simulink model "Gewerk2_Bahnplanung2015"  (Simulink 8.6)
settings: Solver=ode3  StartTime=0.0  StopTime=inf  FixedStep=0.005  RelTol=1e-3
undefined symbols (not defined in the file or in its folder): Com1, none
libraries: xpcrtudplib x9, xpcutilitieslib x5, xpcseriallib x1, slrtlib x1
(part 2 of 2)

== stateflow chart Gewerk2/Chart ==
  state ?
    state Hauptprogramm [parallel]
      settings: executionOrder=1
      state Auftrag_Roboter_1
      state Zielbereich_untersuchen
        entry:
        n4=round((Robbi4_x-528)/400);
        n2=round((Robbi2_x-528)/400);
        n3=round((Robbi3_x-528)/400);
        y2=Robbi2_y;
        y3=Robbi3_y;
        y4=Robbi4_y;
        ersterFifo=floor(Zielstationstation/2)*3+2*mod(Zielstation,2);
      state Uebergabepunkt_gleich_Zielpunkt
        entry:
        for i=1:1:8
        Fifo(i)=0;
        end
        Vektorberechnung=1;
        Auftragskoordinaten=Zielpostion;
      state Fifo_besetzt
        entry:
        Fifobelegt=1;
        zweiterFifo=floor(Zielstation/2)*3+1;
      state Fifo_doppelt_besetzt
        entry:
        dritterFifo=floor(Zielstation/2)*3+2-2*mod(Zielstation,2);
      state Fifo_einfachbesetzt
        entry:
        Vektorberechung=1;
        Auftragskoordinaten=Position(zweiterFifo);
      state Fifo_voll
        entry:
        Vektorberechung=1;
        Auftragskoordinaten=Warteposition;
      state Fifo_doppeltbesetzt
        entry:
        Vektorberechung=1;
        Auftragskoordinaten=Position(driterFifo);
      state AbstandRoboterzumZiel
        entry:
        Abstand=sqrt((Position(Zielstation)(1)-x_ziel1)^2+(y_robotino1-y_ziel1)^2)/100
        ABstände der Roboter zur Zeilstation vergleichen
        anschließend Merker des Fifos zurücksetzten;
      (default) -> Auftrag_Roboter_1
      Auftrag_Roboter_1 -> Zielbereich_untersuchen : [Zielposition>0]
      Zielbereich_untersuchen -> Fifo_besetzt [order 2] : [(ersterFifo==n2| ersterFifo==n3 | ersterFifo==n4)&(y2<=500 | y2<=500 | y2<=500)]
      Zielbereich_untersuchen -> Uebergabepunkt_gleich_Zielpunkt [order 1] : [y2>500 & y3>500 & y4>500]
      Fifo_besetzt -> Fifo_doppelt_besetzt [order 1] : [(zweiterFifo==n2| zweiterFifo==n3 | zweiterFifo==n4)&(y2<=500 | y2<=500 | y2<=500)]
      Fifo_besetzt -> AbstandRoboterzumZiel [order 3] : [(ersterFifo~=n2 & ersterFifo~=n3 & ersterFifo~=n4)]
      Fifo_doppelt_besetzt -> Fifo_voll [order 1] : [(dritterFifo==n2| dritterFifo==n3 | dritterFifo==n4)&(y2<=500 | y2<=500 | y2<=500)]
      Fifo_doppelt_besetzt -> Fifo_besetzt [order 3] : [(zweiterFifo~=n2 & zweiterFifo~=n3 & zweiterFifo~=n4)]
      Fifo_besetzt -> Fifo_einfachbesetzt [order 2]
      Fifo_voll -> Fifo_doppelt_besetzt : [(dritterFifo~=n2 & dritterFifo~=n3 & dritterFifo~=n4)]
      Fifo_doppelt_besetzt -> Fifo_doppeltbesetzt [order 2]
    state Rechnung [parallel]
      during:
      n4=round((Robbi4_x-528)/400);
      n2=round((Robbi2_x-528)/400);
      n3=round((Robbi3_x-528)/400);
      y2=Robbi2_y;
      y3=Robbi3_y;
      y4=Robbi4_y;
      PositionRobbi2=[Robbi2_x Robbi2_y];
      PositionRobbi3=[Robbi2_x Robbi2_y];
      PositionRobbi4=[Robbi2_x Robbi2_y];
      settings: executionOrder=2
    (default) -> Hauptprogramm [order 2]
    (default) -> Rechnung [order 1]
  data: Robbi2_x input double; Robbi3_x input double; Robbi4_x input double; Robbi2_y input double; Robbi3_y input double; Robbi4_y input double; Zielposition input double; Zielstation input double; Vektorberechnung output double; Auftragskoordinaten output double
